simulink model "JONASBROTHERS"  (R2021b)
settings: Solver=FixedStepAuto  StartTime=0.0  StopTime=20  FixedStep=0.0001  RelTol=1e-3
model workspace (MATLAB code in the model file):
  | %% Parameters
  | m_pl = 8800;
  | r_d = 0.2323/2;
  | ig = 4;
  | J_drum = 1.0;
  | J_M = 1.5;
  | %J_M = 2.9;
  | b_hat = 15;
  | 
  | %% Speed Controller
  | t_r = 1e-3;
  | w_BW = log(9)/t_r;
  | %w_BW = 749.6586;
  | w_BWs = 0.1*w_BW;
  | %w_BWs = log(9)/0.09;
  | J_hat = m_pl*((r_d/(ig*4))^2) + J_drum*((1/ig)^2) + J_M
  | 
  | np=2;
  | p=4;
  | i_d_nl = 37.46;
  | %i_d_nl = 65.32;
  | 
  | %% Electrical Parameters
  | R_R_opt = 0.0193;
  | %R_R_opt = 0.04264;
  | R_R_hat = R_R_opt;
  | X_M_opt = 2.81;
  | %X_M_opt = 1.5829;
  | X_sig_opt = 0.0445;
  | %X_sig_opt = 0.0250;
  | omega_rN = 310.5988;
  | omega_N = 314.1593;
  | omega1 = omega_rN;
  | 
  | L_M_hat = X_M_opt/omega1;
  | L_sig_hat = X_sig_opt/omega1;
  | R_s = 0.04264;
  | %R_s = R_R_hat*1.5;
  | %psi_ref = L_M_hat * i_d_nl;
  | psi_ref = 0.8537;
  | %psi_ref = 0.70;
  | KVA = 90/0.85;
  | %V_base = (KVA*1000)/(160*1.73);
  | V_base = 400*sqrt(2)/sqrt(3);
  | alpha_fw = (2*R_R_hat)/L_sig_hat;
  | Ts = 0.0001;
  | I_max = 185;
  | 
  | kps = 2*J_hat*w_BWs/(3*np^2*psi_ref); % notes psi_R_hat is psi_ref
  | kis = w_BWs^2*2*J_hat/(3*np^2*psi_ref); % notes
  | Ba = 2*J_hat/(3*np^2*psi_ref)*(w_BWs-b_hat/J_hat); % notes
  | 
  | kp = w_BW*L_sig_hat;
  | ki = w_BW^2*L_sig_hat;
  | Ra = w_BW*L_sig_hat - (R_R_hat + R_s);
  | R = R_R_hat + R_s;
  | %% Noise
  | sigma_w = 0.5;
  | beta = 10000;
undefined symbols (not defined in the file or in its folder): j, magnitude
libraries: fl_lib x22, nesl_utility x9, CustomComponents_lib x6, simulink x6, slpidlib x2, sdl_lib x1, SignalEditorBlockLib x1
(part 2 of 2)

== matlab function JONASBROTHERS/Indirect Field oriented control/Speed Controller1/MATLAB Function ==
  data: omega_r_ref input size=2; omega_r input size=2; i_q_ref_fw input; I input size=1; w_BWs parameter size=1; i_q_ref output size=2; Inew output; psi_ref parameter size=1; J_hat parameter size=1; Ts parameter; b_hat parameter; I_max parameter; np parameter
function [i_q_ref, Inew]= sc(omega_r_ref, omega_r, i_q_ref_fw,I, w_BWs, psi_ref, J_hat, Ts, b_hat, I_max, np)
%#codegen

%% Speed controller 
% Gains
kps = 2*J_hat*w_BWs/(3*np^2*psi_ref); % notes psi_R_hat is psi_ref
kis = w_BWs^2*2*J_hat/(3*np^2*psi_ref); % notes
ba = 2*J_hat/(3*np^2*psi_ref)*(w_BWs-b_hat/J_hat); % notes
e = omega_r_ref - omega_r;
i_q_ref = kps*e+kis*I-ba*omega_r; % complete: PI + active damping ba, real

%% Update the integral state of the speed controller 
Inew = I + Ts*(e + (i_q_ref_fw - i_q_ref)/kps);

== matlab function JONASBROTHERS/Indirect Field oriented control/Speed Controller1/MATLAB Function1 ==
  data: omega_r_ref input; omega_r input; i_q_ref_fw input; I input size=1; w_BWs parameter size=1; i_q_ref output; Inew output; psi_ref parameter size=1; J_hat parameter size=1; Ts parameter; b_hat parameter; np input
function [i_q_ref, Inew] = sc(omega_r_ref, omega_r, i_q_ref_fw,I, w_BWs, psi_ref, J_hat, Ts, b_hat, np)
%#codegen

%% Current controller 
% Gains
kps = 2*J_hat*w_BWs/(3*np^2*psi_ref);
kis = w_BWs^2*2*J_hat/(3*np^2*psi_ref);
ba = 2*J_hat/(3*np^2*psi_ref)*(w_BWs-b_hat/J_hat);

% 
e = omega_r_ref - omega_r;
i_q_ref = kps*e+kis*I-ba*omega_r; % complete: PI + active damping ba, real

%% Update the integral state of the speed controller 
Inew = I + Ts*(e + (i_q_ref_fw - i_q_ref)/kps);

== matlab function JONASBROTHERS/DrawWork/Wave_Velocity/MATLAB Function ==
  settings: updateMethod=DISCRETE
  data: Hs input; T input; sim_time input; wave output; wave1 output
function [wave, wave1]  = fcn(Hs, T, sim_time)
%WAVE GEN generates stochastic waves
% Hs is the significant wave height [m]
% T is the mean period [s]
% t end is the end time [s]
% t is the time [s]
% wave is sea surface elevation [m]
%% Input parameters
w = linspace (0.1, 2.0, 20); % frequency range
delta_w = w(2) - w(1);
%% PM spectrum (freq. domain )
w1 = (2*pi)/T;
A = 0.11*(Hs^2)*(w1^4);
B = 0.44*(w1^4);
S = (A./w.^5).* exp(-(B./w.^4));
%% Wave amplitude (time domain)
%sfr = 1/25 ; % sampling frequency (Hz) (higher freq −> higher resolution)
t = sim_time; % time vector
phi_test = rng;
phi = 2*pi*(rand(1,length (w))-0.5); % random phase of ith frequency [rad]
rng(phi_test);
A_wave = sqrt(2*S.*delta_w); % amplitude of each sine wave. wave = [] ;

wave1 = [sum(A_wave .*cos(w.*t + phi))];
wave = [sum(A_wave .*-sin(w.*t + phi))];% [m] sea surface elevation  /Derivative

== matlab function JONASBROTHERS/DrawWork/Subsystem/MATLAB Function ==
  data: v input; F_D output
function F_D = fcn(v)
rho = 1025;
C_D = 1.8;
Area_pl = 1.5; 


F_D =sign(-v) * (0.5*rho*v^2*C_D*Area_pl); 
%F_d = 0.5 * cd * rho * A * sign(-v) * v^2;

== matlab function JONASBROTHERS/Load Cases/Case Selector ==
  data: Case1 input; Case2 input; Case3 input; CaseSelector input; payload_ref_pos output
function payload_ref_pos  = fcn(Case1, Case2, Case3, CaseSelector)

if CaseSelector == 1
    payload_ref_pos = Case1;
    %select = "Case 1 in progress";
elseif CaseSelector == 2
    payload_ref_pos = Case2;
    %select = "Case 2 in progress";
elseif CaseSelector == 3
    payload_ref_pos = Case3;
    %select = "Case 3 in progress"; 
else 
    payload_ref_pos = 0;
    %select = "No Case is selected";  
end

== matlab function JONASBROTHERS/DrawWork/MATLAB Function ==
  data: y input; seabed output; v input
function seabed = fcn(y, v)
delta_x = 0 - (y);
k = 1.8e6; % N/m
b = 6.5e5; %Ns/m

if delta_x < 0
    seabed = 0;
elseif delta_x >= 0
    seabed = k*delta_x + b*v*sqrt(delta_x);
else
    seabed = 0;
end

== matlab function JONASBROTHERS/Indirect Field oriented control/Current Controller/MATLAB Function ==
  data: v_sat_dq input size=2; i_s_ref input size=2; i_s input size=2; w_1 input size=1; I input size=1; w_BW parameter size=1; v_s_ref output size=2; Inew output; R_R_hat parameter size=1; L_sig_hat parameter size=1; Ts parameter; R_s input
function [v_s_ref, Inew] = cc(v_sat_dq,i_s_ref, i_s, w_1, I, w_BW, R_R_hat, L_sig_hat, Ts, R_s)
%#codegen

%% Current controller 
% Gains
kp = w_BW*L_sig_hat; % L7 p15
ki = w_BW^2*L_sig_hat; % L7 p15
Ra = w_BW*L_sig_hat - (R_R_hat + R_s); % L7 p14(R_R_hat+R_s)

% Voltage reference in synchronous coordinates
i_s = i_s(1)+ 1i*i_s(2);
i_s_ref = i_s_ref(1)+ 1i*i_s_ref(2);
e = i_s_ref - i_s;
% L7 p13 and p15 (c for complex number)
v_s_ref_c = kp*e+ki*I + 1i*w_1*L_sig_hat*i_s_ref-Ra*i_s_ref; % complete: PI + active resistance Ra + decoupler.
v_s_ref = [real(v_s_ref_c);imag(v_s_ref_c)];

%% Update the integral state of the current controller 
v_sat_dq_c = v_sat_dq(1)+ 1i*v_sat_dq(2);
Inew = I + Ts*(e + (v_sat_dq_c)/kp);

== matlab function JONASBROTHERS/Indirect Field oriented control/dq->abc/MATLAB Function ==
  data: vs_dq input size=2; thetas input size=1; vs_abc output size=3
function vs_abc = dq_abc(vs_dq, thetas)
%#codegen

% voltage in synchronous coordinates:
 vd = vs_dq(1); vq = vs_dq(2); 
vs_dq = [vd;vq];

% coordinate transformation and Space-vector transformation 
T_alphabeta = [cos(thetas), -sin(thetas); sin(thetas), cos(thetas)];
T_23 = [1, 0; -1/2, sqrt(3)/2; -1/2, -sqrt(3)/2];
vs_abc = T_23*T_alphabeta*vs_dq;   % Complete this

== matlab function JONASBROTHERS/Indirect Field oriented control/abc->dq1/MATLAB Function ==
  data: is_abc input size=3; thetas input size=1; is output size=2
function is = abc_dq(is_abc, thetas)
%#codegen

% Phase currents
ia = is_abc(1); ib = is_abc(2); ic = is_abc(3); 
is_abc = [ia;ib;ic];
% Space-vector transformation and coordinate transformation
T_dq = [cos(thetas), sin(thetas); -sin(thetas), cos(thetas)];
T_32 = [2/3, -1/3, -1/3; 0, 1/sqrt(3), -1/sqrt(3)];
is = T_dq*T_32*is_abc;   % Complete this
